simulink model "controller_block"  (R2014b)
settings: Solver=ode45  StartTime=0.0  StopTime=10.0  RelTol=1e-3
values from neighbouring files (symbols this model uses):
  operating_q = [0 0 0 0 0 0 0 0 0 0 0 0]'    [main.m]
  Qu = diag([5 5 5 5])    [main.m]
  Qx = 1e-1*diag([0.1 0.1 0.1 0.1 0.1 0.1 100 100 100 0.1 0.1 0.1])    [main.m]
undefined symbols (not defined in the file or in its folder): Engine_back, Engine_front, Engine_left, Engine_right, operating_u
settings Model: Creator=Abhiram  LastModifiedBy=Abhiram

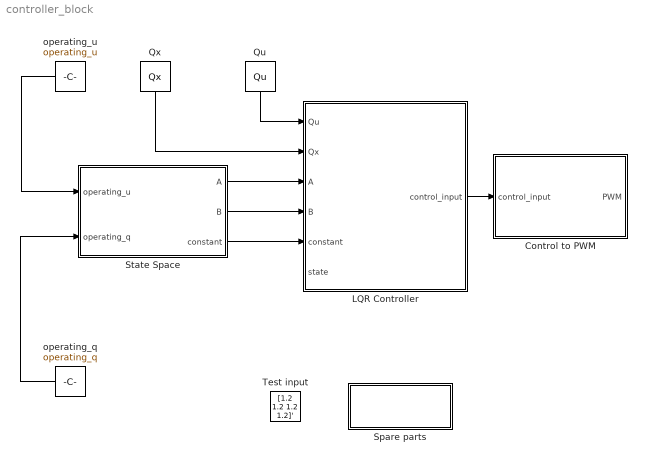
== system controller_block ==
  Control to PWM : MATLAB Function  TreatAsAtomicUnit=on
  LQR Controller : MATLAB Function  TreatAsAtomicUnit=on
  Qu : Constant  Value=Qu
  Qx : Constant  Value=Qx
  Spare parts : Subsystem
  State Space : MATLAB Function  TreatAsAtomicUnit=on
  Test input : Constant  Value=[1.2 1.2 1.2 1.2]'
  operating_q : Constant  Value=operating_q
  operating_u : Constant  Value=operating_u
  wires:
  State Space/1(A) -> LQR Controller/3(A)
  State Space/2(B) -> LQR Controller/4(B)
  State Space/3(constant) -> LQR Controller/5(constant)
  Qx/1 -> LQR Controller/2(Qx)
  Qu/1 -> LQR Controller/1(Qu)
  LQR Controller/1(control_input) -> Control to PWM/1(control_input)
  operating_u/1 -> State Space/1(operating_u)
  operating_q/1 -> State Space/2(operating_q)

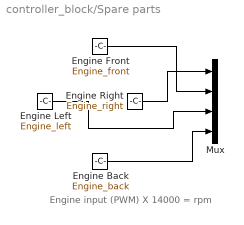
== system controller_block/Spare parts ==
  note: Engine input (PWM) X 14000 = rpm
  Engine Back : Constant  Value=Engine_back
  Engine Front : Constant  Value=Engine_front
  Engine Left : Constant  Value=Engine_left
  Engine Right : Constant  Value=Engine_right
  Mux : Mux
  wires:
  Engine Right/1 -> Mux/1
  Engine Front/1 -> Mux/2
  Engine Left/1 -> Mux/3
  Engine Back/1 -> Mux/4

== matlab function controller_block/State Space ==
  data: operating_u input; operating_q input; A output; B output; constant output
function [A, B, constant] = fcn(operating_u, operating_q)
% function [A, B, constant] = fcn(operating_u, operating_q)
% function [A, B, constant] = fcn(operating_u, operating_q)
% 
% Ixx = 2.09*10^(-05);
% Iyy = 2.09*10^(-05);
% Izz = 3.81*10^(-05);
% d = 0.046;
% m = 0.027;
% g = 9.8;
% 
% theta_0 = operating_q(1);
% phi_0 = operating_q(2);
% psi_0 = operating_q(3);
% theta_dot_0 = operating_q(4);
% phi_dot_0 = operating_q(5);
% psi_dot_0 = operating_q(6);
% x_0 = operating_q(7);
% y_0 = operating_q(8);
% z_0 = operating_q(9);
% x_dot_0 = operating_q(10);
% y_dot_0 = operating_q(11);
% z_dot_0 = operating_q(12);
% 
% f_0 = operating_u(1);                                                       % Thrust
% T_theta_0 = operating_u(1);                                                 % Pitch torque
% T_phi_0 = operating_u(2);                                                   % Roll Torque
% T_psi_0 = operating_u(3);                                                   % Yaw Torque
% 
% % Assignment for simplification
% wx_0 = theta_dot_0;
% wy_0 = phi_dot_0;
% wz_0 = psi_dot_0;
% 
% A_trans = (1/m)*[ -f_0*cos(theta_0),                             0,             0;
%                   -f_0*sin(theta_0)*sin(phi_0),  f_0*cos(theta_0)*cos(phi_0),   0;
%                   -f_0*sin(theta_0)*cos(phi_0), -f_0*cos(theta_0)*sin(phi_0),   0];
%           
% B_trans = (1/m)*[ -sin(theta_0); cos(theta_0)*sin(phi_0); cos(theta_0)*cos(phi_0) ];
% 
% K_trans = (1/m)*[ f_0*theta_0*cos(theta_0);
%                   f_0*sin(theta_0)*sin(phi_0)*theta_0 - f_0*cos(theta_0)*cos(phi_0)*phi_0;
%                   f_0*sin(theta_0)*cos(phi_0)*theta_0 + f_0*cos(theta_0)*sin(phi_0)*phi_0 - m*g];
% 
% A_angle = [  0,                  -wz_0*(Izz - Iyy)/Ixx,  -wy_0*(Izz - Iyy)/Ixx;
%             -wz_0*(Ixx - Izz)/Iyy,   0,                  -wx_0*(Ixx - Izz)/Iyy;
%             -wy_0*(Iyy - Ixx)/Izz,  -wx_0*(Iyy - Ixx)/Izz,   0                ];
%         
% B_angle = [ (1/Ixx),    0,        0;
%              0,      (1/Iyy),     0;
%              0,         0,      (1/Izz)];
% 
% K_angle = [ wy_0*wz_0*(Izz - Iyy)/Ixx;    wx_0*wz_0*(Ixx- Izz)/Iyy;    wx_0*wy_0*(Iyy - Ixx)/Izz];
% 
% % vector Sequence - angles_pitch.roll.yaw,angles_dot,translation_x.y.z, translation_dot
% 
% A = [ zeros(3,3),   eye(3),      zeros(3,3),  zeros(3,3);
%       zeros(3,3),   A_angle,     zeros(3,3),  zeros(3,3);
%       zeros(3,3),   zeros(3,3),  zeros(3,3),  eye(3);
%       A_trans,      zeros(3,3),  zeros(3,3),  zeros(3,3)];
% 
% B = [ zeros(3,4);
%       zeros(3,1), B_angle;
%       zeros(3,4);
%       B_trans, zeros(3,3)];
% 
% constant = [ zeros(3,1);
%              K_angle;
%              zeros(3,1);
%              K_trans];
% end

== matlab function controller_block/LQR Controller ==
  data: Qu input; control_input output; Qx input; A input; B input; constant input; state input
function control_input = fcn(Qu, Qx, A, B, constant, state)
% function control_input = fcn(Qu, Qx, A, B, constant, state)
% 
% coder.extrinsic('lqr');
% Klqr = lqr(A,B,Qx,Qu);
% 
% control_input = -Klqr*(state + A\constant);
% 
% control_input = -Klqr*(state);
% control_input = 0;A
% 
% end

== matlab function controller_block/Control to PWM ==
  data: control_input input; PWM output
function PWM = fcn(control_input)
% function PWM = fcn(control_input)
% function PWM  = fcn(control_input)
% % Provides PWM signal for perticular control input
% 
% Ct = 1.0942e-07;
% C1 = 0.25*(Ct)*9.8/1000;                                                    % grams to newton                           
% Cq = 1*(10^(-9))*(60/(2*pi))^2;                                             % Cq in rpm
% d = 0.046;
% 
% Kv =  14000*[1 0 0 0
%              0 1 0 0
%              0 0 1 0
%              0 0 0 1]';
% 
% B = control_input;
% 
% A = [  C1   C1    C1    C1;
%        0    d*C1  0    -d*C1;
%       -d*C1 0     d*C1  0;
%       -Cq   Cq   -Cq    Cq];
% 
% X = linsolve(A,B);
% 
% w1 = sqrt(X(1));
% w2 = sqrt(X(2));
% w3 = sqrt(X(3));
% w4 = sqrt(X(4));
% 
% PWM = Kv\[w1; w2; w3; w4];
% 
% end
